simulink library "pressure_drop_for_measured_data_water"  (R2018b)
settings: Solver=ode45  StartTime=0.0  StopTime=10.0  RelTol=1e-3  EnableMultiTasking=on
undefined symbols (not defined in the file): acol
settings Model: Creator=lena.frank  LastModifiedBy=drhf
settings DataIOCC: LimitDataPoints=on  SaveFormat=Array  SignalLoggingSaveFormat=ModelDataLogs
settings OptimizationCC: ExpressionDepthLimit=2147483647  LifeSpan=inf
settings DebuggingCC: UnderspecifiedInitializationDetection=Classic  MergeDetectMultiDrivingBlocksExec=none  SolverPrmCheckMsg=warning  FcnCallInpInsideContextMsg=warning  StateNameClashWarn=warning  SFUnexpectedBacktrackingDiag=warning  SFNoUnconditionalDefaultTransitionDiag=warning  SFExecutionAtInitializationDiag=none
settings HardwareCC: ProdBitPerPointer=32  ProdBitPerSizeT=32  ProdBitPerPtrDiffT=32  ProdLargestAtomicFloat=None  ProdIntDivRoundTo=Undefined  ProdEndianess=Unspecified  ProdWordSize=32  ProdHWDeviceType=32-bit Generic
settings ModelReferenceCC: PropagateSignalLabelsOutOfModel=off
settings SFSimCC: SimUseLocalCustomCode=off
settings RTWCC: RTWUseLocalCustomCode=off
settings CodeAppCC: StateflowObjectComments=on
settings GRTTargetCC: TargetLangStandard=C89/C90 (ANSI)  GeneratePreprocessorConditionals=Disable all  CombineOutputUpdateFcns=off  GRTInterface=on
settings ConfigComp: CovMetricSettings=dw  CovHtmlReporting=on  CovSaveCumulativeToWorkspaceVar=on  CovSaveSingleToWorkspaceVar=on  CovExternalEMLEnable=off

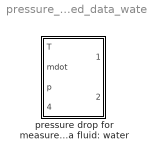
== system pressure_drop_for_measured_data_water ==
  pressure drop for measured data fluid: water : Subsystem  mask(pressure drop measured data, fluid water){mdottest=0.01*1.96, ttest=20, pdroptest=158*1.96, aonecol=1.96, acol=acol}
      mask prompts: mdottest "massflow at test condition condition [kg/s]"; ttest "temperature at test condition [degree centigrade]"; pdroptest "pressure drop in test [Pa]"; aonecol "surface of one collector [m²]"; acol "total surface of array (DO NOT CHANGE HERE)"
      mask help:
      | This block calculates the pressure drop of a collector from measured data.
      | Other massflow rates and temperatures than at test condition are interpolated according to a typical massflow to pressure drop correlation of a collector for the fluid water.
      | Set "surface of one collector" to the surface of one collector for a parallel arrangement of collectors. Set it to the surface of the array "acol" to model a series arrangement.
      mask Help: web(fullfile(path_carnot('help'),'pressure_drop_for_measured_data_water.html'),'-helpbrowser')

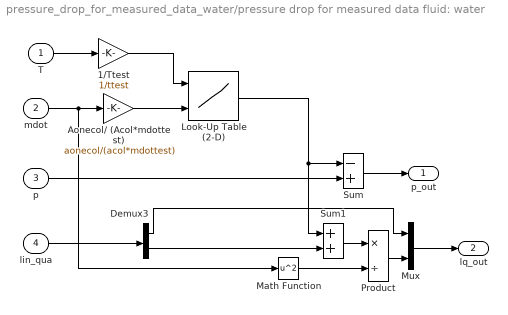
== system pressure_drop_for_measured_data_water/pressure drop for measured data fluid: water ==
  T : Inport
  mdot : Inport  Port=2
  p : Inport  Port=3
  lin_qua : Inport  Port=4
  1/Ttest : Gain  Gain=1/ttest  SaturateOnIntegerOverflow=on  OutDataTypeStr=Inherit: Same as input  ParamDataTypeStr=Inherit: Same as input
  Aonecol/ (Acol*mdottest) : Gain  Gain=aonecol/(acol*mdottest)  SaturateOnIntegerOverflow=on  OutDataTypeStr=Inherit: Same as input  ParamDataTypeStr=Inherit: Same as input
  Demux3 : Demux  Outputs=2
  Look-Up Table (2-D) : Lookup2D  RowIndex=0:2.5:10  ColumnIndex=0:0.6175:3.0875  Table="pdroptest*[0  0.7699  1.6541  2.6516  3.7617  4.9841;  0  0.28  0.674  1.1811  1.8007  2.5325;  0  0.1889  0.4946  0.9163  1.4532  2.1052;  0  0.1532  0.4284  0.8243  1.3406  1.9767;  0  0.1372  0.4056  0.8042  1.3323  1.9896]"  SaturateOnIntegerOverflow=on  InputSameDT=on
  Math Function : Math  Operator=square  SaturateOnIntegerOverflow=on
  Mux : Mux  Inputs=2
  Product : Product  Inputs=*/  SaturateOnIntegerOverflow=on  InputSameDT=on  OutDataTypeStr=Inherit: Same as first input
  Sum : Sum  Inputs=-+  SaturateOnIntegerOverflow=on  InputSameDT=on  OutDataTypeStr=Inherit: Same as first input
  Sum1 : Sum  SaturateOnIntegerOverflow=on  InputSameDT=on  OutDataTypeStr=Inherit: Same as first input
  p_out : Outport
  lq_out : Outport  Port=2
  wires:
  mdot/1 -> Math Function/1, Aonecol/ (Acol*mdottest)/1
  Look-Up Table (2-D)/1 -> Sum1/1, Sum/1
  p/1 -> Sum/2
  Sum/1 -> p_out/1
  Demux3/1 -> Mux/1
  Mux/1 -> lq_out/1
  Product/1 -> Mux/2
  Math Function/1 -> Product/2
  Sum1/1 -> Product/1
  Demux3/2 -> Sum1/2
  lin_qua/1 -> Demux3/1
  T/1 -> 1/Ttest/1
  1/Ttest/1 -> Look-Up Table (2-D)/1
  Aonecol/ (Acol*mdottest)/1 -> Look-Up Table (2-D)/2
